simulink model "mophong_quy_dao"  (R2015a)
settings: Solver=ode45  StartTime=0.0  StopTime=322  RelTol=1e-3
values from neighbouring files (symbols this model uses):
  s = [s; t E]    [quydao.m]
undefined symbols (not defined in the file or in its folder): lap, RootGround, RootPart
libraries: mblibv1 x17
settings Model: Creator=Administrator  LastModifiedBy=Administrator
settings SimMechanicsCC: VisOnUpdateDiagram=on  VisDuringSimulation=on

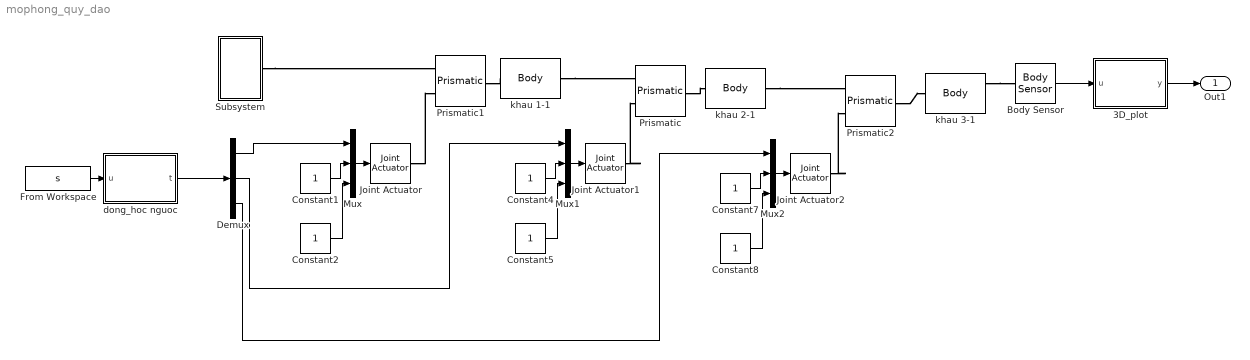
== system mophong_quy_dao ==
  3D_plot : MATLAB Function  TreatAsAtomicUnit=on
  Body Sensor : mblibv1/Sensors &  Actuators/Body Sensor  UpdateFromCAD=off  PhysicalDomain=Mechanical  PortType=blob  Muxed=on  Pose=off  Angle=on  AngleUnits=deg  ArcVelocity=off  ArcVelocityUnits=deg/s  ArcAcceleration=off  ArcAccelerationUnits=deg/s^2  CoordPosition=on  CoordPositionUnits=mm  Velocity=off  VelocityUnits=m/s  Acceleration=off  AccelerationUnits=m/s^2  Quaternion=on  QuaternionDT=off  QuaternionDDT=off  QuaternionUnits=off  OutputVector=[1]  ActiveIO=on  Width=3  DialogClass=MechanicalSensorBlock  ReferenceFrame=Absolute (World)
  Constant{1..2,4..5,7..8} (6 alike) : Constant
  Demux : Demux  Outputs=3
  From Workspace : FromWorkspace  VariableName=s  SampleTime=0.4
  Joint Actuator : mblibv1/Sensors &  Actuators/Joint Actuator  UpdateFromCAD=off  PhysicalDomain=Mechanical  PortType=blob  ActuationStyle=Motion  AngleUnits=deg  ArcVelocityUnits=deg/s  ArcAccelerationUnits=deg/s^2  CoordPositionUnits=mm  VelocityUnits=m/s  AccelerationUnits=m/s^2  ForceUnits=N  TorqueUnits=N*m  ActiveIO=on  Width=3  DialogClass=MechanicalActuatorBlock  Primitive=P1  ReferenceFrame=Absolute (World)
  Joint Actuator1 : mblibv1/Sensors &  Actuators/Joint Actuator  UpdateFromCAD=off  PhysicalDomain=Mechanical  PortType=blob  ActuationStyle=Motion  AngleUnits=deg  ArcVelocityUnits=deg/s  ArcAccelerationUnits=deg/s^2  CoordPositionUnits=mm  VelocityUnits=m/s  AccelerationUnits=m/s^2  ForceUnits=N  TorqueUnits=N*m  ActiveIO=on  Width=3  DialogClass=MechanicalActuatorBlock  Primitive=P1  ReferenceFrame=Absolute (World)
  Joint Actuator2 : mblibv1/Sensors &  Actuators/Joint Actuator  UpdateFromCAD=off  PhysicalDomain=Mechanical  PortType=blob  ActuationStyle=Motion  AngleUnits=deg  ArcVelocityUnits=deg/s  ArcAccelerationUnits=deg/s^2  CoordPositionUnits=mm  VelocityUnits=m/s  AccelerationUnits=m/s^2  ForceUnits=N  TorqueUnits=N*m  ActiveIO=on  Width=3  DialogClass=MechanicalActuatorBlock  Primitive=P1  ReferenceFrame=Absolute (World)
  Mux : Mux  Inputs=3
  Mux1 : Mux  Inputs=3
  Mux2 : Mux  Inputs=3
  Prismatic : mblibv1/Joints/Prismatic  LConnTagsString=__newl0|SA1  RConnTagsString=__newr0  UpdateFromCAD=on  PMImportedID=khau 1-1:-:khau 2-1  NumSAPorts=1  CutJoint=off  MarkAsCut=off  Primitives=prismatic  PrimitiveProps=P1$World$[-1,0,0]$prismatic  DialogClass=JointBlock  P1Axis=[-1,0,0]
  Prismatic1 : mblibv1/Joints/Prismatic  LConnTagsString=__newl0|SA1  RConnTagsString=__newr0  UpdateFromCAD=on  PMImportedID=khau 0-1:-:khau 1-1  NumSAPorts=1  CutJoint=off  MarkAsCut=off  Primitives=prismatic  PrimitiveProps=P1$World$[0,0,1]$prismatic  DialogClass=JointBlock  P1Axis=[0,0,1]
  Prismatic2 : mblibv1/Joints/Prismatic  LConnTagsString=__newl0|SA1  RConnTagsString=__newr0  UpdateFromCAD=on  PMImportedID=khau 2-1:-:khau 3-1  NumSAPorts=1  CutJoint=off  MarkAsCut=off  Primitives=prismatic  PrimitiveProps=P1$World$[0,-1,0]$prismatic  DialogClass=JointBlock  P1Axis=[0,-1,0]
  Subsystem : Subsystem
  dong_hoc nguoc : MATLAB Function  TreatAsAtomicUnit=on
  khau 1-1 : mblibv1/Bodies/Body  LConnTagsString=CS3  RConnTagsString=CS2  UpdateFromCAD=on  PMImportedID=khau 1-1  DialogClass=MechanicalBodyBlock  Mass=0.0250848  MassUnits=kg  InertiaUnits=kg*m^2  Inertia=[0.000583644,0,0;0,0.000587076,0;0,0,3.56803e-05]  Shape=Cylinder  ShapeDims=[1 1]  ShapeUnits=m  ShapeUse=false  Density=1  DensityUnits=kg/m^3  DensityUse=false  GraphicsMode=GFXFILE  GraphicsFileName=lap - khau 1-1.STL  BodyColorSelMode=COLORPALETTE  BodyColor=[0;0.501961;1]  AttachedToCS=CS1  CG=Right$CG$[0.225672 0 0.06]$WORLD$WORLD$m$[0 0 1;-1 0 0;0 -1 0]$3x3 Transform$rad$WORLD$false$khau 1-1::CG(AUTOGEN)  WorkingFrames=Right$CS1$[0 0 0.06]$WORLD$WORLD$m$[0 0 1;-1 0 0;0 -1 0]$3x3 Transform$rad$WORLD$false$khau 1-1::CS1(AUTOGEN)#Right$CS2$[0.48 -0.04 0.1]$WORLD$WORLD$m$[1 0 0;0 1 0;0 0 1]$3x3 Transform$rad$WORLD$true$khau 1-1:-:khau 2-1::khau 1-1(AUTOGEN)#Left$CS3$[-0.05 0.05 0.12]$WORLD$WORLD$m$[1 0 0;0 1 0;0 0 1]$3x3 Transform$rad$WORLD$true$khau 0-1:-:khau 1-1::khau 1-1(AUTOGEN)  CGPos=[0.225672 0 0.06]  CGRot=[0 0 1;-1 0 0;0 -1 0]  CS0Pos=[]  CS0Rot=[]  CS1Pos=[0 0 0.06]  CS1Rot=[0 0 1;-1 0 0;0 -1 0]  CS2Pos=[0.48 -0.04 0.1]  CS2Rot=[1 0 0;0 1 0;0 0 1]  CS3Pos=[-0.05 0.05 0.12]  CS3Rot=[1 0 0;0 1 0;0 0 1]  CS4Pos=[]  CS4Rot=[]  CS5Pos=[]  CS5Rot=[]  CS6Pos=[]  CS6Rot=[]  CS7Pos=[]  CS7Rot=[]  CS8Pos=[]  CS8Rot=[]  CS9Pos=[]  CS9Rot=[]  CS10Pos=[]  CS10Rot=[]  CS11Pos=[]  CS11Rot=[]  CS12Pos=[]  CS12Rot=[]  CS13Pos=[]  CS13Rot=[]  CS14Pos=[]  CS14Rot=[]  CS15Pos=[]  CS15Rot=[]  CS16Pos=[]  CS16Rot=[]  CS17Pos=[]  CS17Rot=[]  CS18Pos=[]  CS18Rot=[]  CS19Pos=[]  CS19Rot=[]  CS20Pos=[]  CS20Rot=[]
  khau 2-1 : mblibv1/Bodies/Body  LConnTagsString=CS2  RConnTagsString=CS3  UpdateFromCAD=on  PMImportedID=khau 2-1  DialogClass=MechanicalBodyBlock  Mass=0.0401856  MassUnits=kg  InertiaUnits=kg*m^2  Inertia=[0.00271366,0,0;0,0.00271765,0;0,0,7.5687e-05]  Shape=Cylinder  ShapeDims=[1 1]  ShapeUnits=m  ShapeUse=false  Density=1  DensityUnits=kg/m^3  DensityUse=false  GraphicsMode=GFXFILE  GraphicsFileName=lap - khau 2-1.STL  BodyColorSelMode=COLORPALETTE  BodyColor=[0.901961;0.709804;0.439216]  AttachedToCS=CS1  CG=Right$CG$[0.42 -0.0425466 0.06]$WORLD$WORLD$m$[0 1 0;0 0 -1;-1 0 0]$3x3 Transform$rad$WORLD$false$khau 2-1::CG(AUTOGEN)  WorkingFrames=Right$CS1$[0.42 0 0.06]$WORLD$WORLD$m$[0 1 0;0 0 -1;-1 0 0]$3x3 Transform$rad$WORLD$false$khau 2-1::CS1(AUTOGEN)#Left$CS2$[0.32 -0.04 0.1]$WORLD$WORLD$m$[1 0 0;0 1 0;0 0 1]$3x3 Transform$rad$WORLD$true$khau 1-1:-:khau 2-1::khau 2-1(AUTOGEN)#Right$CS3$[0.395 -0.06 0.085]$WORLD$WORLD$m$[1 0 0;0 1 0;0 0 1]$3x3 Transform$rad$WORLD$true$khau 2-1:-:khau 3-1::khau 2-1(AUTOGEN)  CGPos=[0.42 -0.0425466 0.06]  CGRot=[0 1 0;0 0 -1;-1 0 0]  CS0Pos=[]  CS0Rot=[]  CS1Pos=[0.42 0 0.06]  CS1Rot=[0 1 0;0 0 -1;-1 0 0]  CS2Pos=[0.32 -0.04 0.1]  CS2Rot=[1 0 0;0 1 0;0 0 1]  CS3Pos=[0.395 -0.06 0.085]  CS3Rot=[1 0 0;0 1 0;0 0 1]  CS4Pos=[]  CS4Rot=[]  CS5Pos=[]  CS5Rot=[]  CS6Pos=[]  CS6Rot=[]  CS7Pos=[]  CS7Rot=[]  CS8Pos=[]  CS8Rot=[]  CS9Pos=[]  CS9Rot=[]  CS10Pos=[]  CS10Rot=[]  CS11Pos=[]  CS11Rot=[]  CS12Pos=[]  CS12Rot=[]  CS13Pos=[]  CS13Rot=[]  CS14Pos=[]  CS14Rot=[]  CS15Pos=[]  CS15Rot=[]  CS16Pos=[]  CS16Rot=[]  CS17Pos=[]  CS17Rot=[]  CS18Pos=[]  CS18Rot=[]  CS19Pos=[]  CS19Rot=[]  CS20Pos=[]  CS20Rot=[]
  khau 3-1 : mblibv1/Bodies/Body  LConnTagsString=CS2  RConnTagsString=CG|CS1  UpdateFromCAD=on  PMImportedID=khau 3-1  DialogClass=MechanicalBodyBlock  Mass=0.00253036  MassUnits=kg  InertiaUnits=kg*m^2  Inertia=[3.10671e-06,0,0;0,4.33218e-06,0;0,0,3.82518e-06]  Shape=Cylinder  ShapeDims=[1 1]  ShapeUnits=m  ShapeUse=false  Density=1  DensityUnits=kg/m^3  DensityUse=false  GraphicsMode=GFXFILE  GraphicsFileName=lap - khau 3-1.STL  BodyColorSelMode=COLORPALETTE  BodyColor=[0.28628 0.66275 0.32941]  AttachedToCS=CS1  CG=Right$CG$[0.416709 -0.66 0.06]$WORLD$WORLD$m$[-1 0 0;0 1 0;0 0 -1]$3x3 Transform$rad$WORLD$true$khau 3-1::CG(AUTOGEN)  WorkingFrames=Right$CS1$[0.31 -0.66 0.06]$WORLD$WORLD$m$[-1 0 0;0 1 0;0 0 -1]$3x3 Transform$rad$WORLD$true$khau 3-1::CS1(AUTOGEN)#Left$CS2$[0.395 -0.72 0.085]$WORLD$WORLD$m$[1 0 0;0 1 0;0 0 1]$3x3 Transform$rad$WORLD$true$khau 2-1:-:khau 3-1::khau 3-1(AUTOGEN)  CGPos=[0.416709 -0.66 0.06]  CGRot=[-1 0 0;0 1 0;0 0 -1]  CS0Pos=[]  CS0Rot=[]  CS1Pos=[0.31 -0.66 0.06]  CS1Rot=[-1 0 0;0 1 0;0 0 -1]  CS2Pos=[0.395 -0.72 0.085]  CS2Rot=[1 0 0;0 1 0;0 0 1]  CS3Pos=[]  CS3Rot=[]  CS4Pos=[]  CS4Rot=[]  CS5Pos=[]  CS5Rot=[]  CS6Pos=[]  CS6Rot=[]  CS7Pos=[]  CS7Rot=[]  CS8Pos=[]  CS8Rot=[]  CS9Pos=[]  CS9Rot=[]  CS10Pos=[]  CS10Rot=[]  CS11Pos=[]  CS11Rot=[]  CS12Pos=[]  CS12Rot=[]  CS13Pos=[]  CS13Rot=[]  CS14Pos=[]  CS14Rot=[]  CS15Pos=[]  CS15Rot=[]  CS16Pos=[]  CS16Rot=[]  CS17Pos=[]  CS17Rot=[]  CS18Pos=[]  CS18Rot=[]  CS19Pos=[]  CS19Rot=[]  CS20Pos=[]  CS20Rot=[]
  Out1 : Outport
  wires:
  Demux/1 -> Mux/1
  Constant1/1 -> Mux/2
  Constant2/1 -> Mux/3
  Mux/1 -> Joint Actuator/1
  Demux/2 -> Mux1/1
  Constant4/1 -> Mux1/2
  Constant5/1 -> Mux1/3
  Mux1/1 -> Joint Actuator1/1
  Demux/3 -> Mux2/1
  Constant7/1 -> Mux2/2
  Constant8/1 -> Mux2/3
  Mux2/1 -> Joint Actuator2/1
  dong_hoc nguoc/1(t) -> Demux/1
  Body Sensor/1 -> 3D_plot/1(u)
  3D_plot/1(y) -> Out1/1
  From Workspace/1 -> dong_hoc nguoc/1(u)
  connections:
  khau 1-1/RConn1 -- Prismatic/LConn1
  Prismatic/RConn1 -- khau 2-1/LConn1
  Prismatic1/RConn1 -- khau 1-1/LConn1
  khau 2-1/RConn1 -- Prismatic2/LConn1
  Prismatic2/RConn1 -- khau 3-1/LConn1
  Joint Actuator/RConn1 -- Prismatic1/LConn2
  Joint Actuator1/RConn1 -- Prismatic/LConn2
  Joint Actuator2/RConn1 -- Prismatic2/LConn2
  khau 3-1/RConn1 -- Body Sensor/LConn1
  Subsystem/RConn1 -- Prismatic1/LConn1

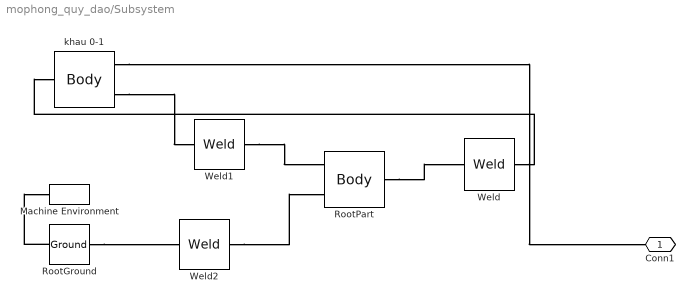
== system mophong_quy_dao/Subsystem ==
  Machine Environment : mblibv1/Bodies/Machine Environment  PortType=env  PhysicalDomain=Mechanical  DialogTemplateClass=MECH.MachineEnvironment  SyncWhenCopied=off  Gravity=[0 -9.81 0]  GravityUnits=m/s^2  GravityAsSignal=off  Dimensionality=Auto-detect  AnalysisType=Forward dynamics  LinearAssemblyTolerance=1e-3  LinearAssemblyToleranceUnits=m  AngularAssemblyTolerance=1e-3  AngularAssemblyToleranceUnits=rad  ConstraintSolverType=Stabilizing  ConstraintRelTolerance=1e-4  ConstraintAbsTolerance=1e-4  UseRobustSingularityHandling=off  RedundancyAnalysisToleranceType=Automatically select tolerance  RedundancyAnalysisTolerance=1e-14  StatePerturbationType=Fixed  PerturbationSize=1e-5  VisualizeMachine=on  BodyVisualizationType=Use model default body geometries  BodyColorSelMode=Use model default  DefaultBodyColor=[1 0 0]
  RootGround : mblibv1/Bodies/Ground  UpdateFromCAD=on  PMImportedID=RootGround  LeftPortType=env  RightPortType=workingframe  PhysicalDomain=Mechanical  DialogClass=GroundBlock  CoordPosition=[0.0188363,-0.0133914,0.352544]  CoordPositionUnits=m  StateVectorMgrId=0  MachineId=[1 0]  ShowEnvPort=on  ParameterChecksum=[2388317299, 529211876, 2012815551, 1180572592]  TopologyChecksum=[3572386912, 2938984299, 652651862, 2599928849]
  RootPart : mblibv1/Bodies/Body  LConnTagsString=CS3|CS4  RConnTagsString=CS2  UpdateFromCAD=on  PMImportedID=lap/RootPart  DialogClass=MechanicalBodyBlock  Mass=0  MassUnits=kg  InertiaUnits=kg*m^2  Inertia=[0,0,0;0,0,0;0,0,0]  Shape=Cylinder  ShapeDims=[1 1]  ShapeUnits=m  ShapeUse=false  Density=1  DensityUnits=kg/m^3  DensityUse=false  GraphicsMode=MACHINE_DEFAULT  BodyColorSelMode=MACHINE_DEFAULT  BodyColor=[1;0;0]  AttachedToCS=CS1  CG=Right$CG$[0.0188363 -0.0133914 0.352544]$WORLD$WORLD$m$[1 0 0;0 1 0;0 0 1]$3x3 Transform$rad$WORLD$false$lap/RootPart::CG(AUTOGEN)  WorkingFrames=Right$CS1$[0 0 0]$WORLD$WORLD$m$[1 0 0;0 1 0;0 0 1]$3x3 Transform$rad$WORLD$false$lap/RootPart::CS1(AUTOGEN)#Right$CS2$[-0.102063 0 0.46]$WORLD$WORLD$m$[1 0 0;0 1 0;0 0 1]$3x3 Transform$rad$WORLD$true$khau 0-1:-:lap/RootPart::lap/RootPart(AUTOGEN)#Left$CS3$[-0.102063 0 0.46]$WORLD$WORLD$m$[1 0 0;0 1 0;0 0 1]$3x3 Transform$rad$WORLD$true$:-:khau 0-1::lap/RootPart(AUTOGEN)#Left$CS4$[0.0188363 -0.0133914 0.352544]$WORLD$WORLD$m$[1 0 0;0 1 0;0 0 1]$3x3 Transform$rad$WORLD$true$RootGround:-:lap/RootPart::lap/RootPart(AUTOGEN)  CGPos=[0.0188363 -0.0133914 0.352544]  CGRot=[1 0 0;0 1 0;0 0 1]  CS0Pos=[]  CS0Rot=[]  CS1Pos=[0 0 0]  CS1Rot=[1 0 0;0 1 0;0 0 1]  CS2Pos=[-0.102063 0 0.46]  CS2Rot=[1 0 0;0 1 0;0 0 1]  CS3Pos=[-0.102063 0 0.46]  CS3Rot=[1 0 0;0 1 0;0 0 1]  CS4Pos=[0.0188363 -0.0133914 0.352544]  CS4Rot=[1 0 0;0 1 0;0 0 1]  CS5Pos=[]  CS5Rot=[]  CS6Pos=[]  CS6Rot=[]  CS7Pos=[]  CS7Rot=[]  CS8Pos=[]  CS8Rot=[]  CS9Pos=[]  CS9Rot=[]  CS10Pos=[]  CS10Rot=[]  CS11Pos=[]  CS11Rot=[]  CS12Pos=[]  CS12Rot=[]  CS13Pos=[]  CS13Rot=[]  CS14Pos=[]  CS14Rot=[]  CS15Pos=[]  CS15Rot=[]  CS16Pos=[]  CS16Rot=[]  CS17Pos=[]  CS17Rot=[]  CS18Pos=[]  CS18Rot=[]  CS19Pos=[]  CS19Rot=[]  CS20Pos=[]  CS20Rot=[]
  Weld : mblibv1/Joints/Weld  LConnTagsString=__newl0  RConnTagsString=__newr0  UpdateFromCAD=on  PMImportedID=khau 0-1:-:lap/RootPart  NumSAPorts=0  CutJoint=off  MarkAsCut=off  Primitives=weld  PrimitiveProps=W$World$[0.57735,0.57735,0.57735]$weld  DialogClass=JointBlock  WAxis=[0.57735,0.57735,0.57735]
  Weld1 : mblibv1/Joints/Weld  LConnTagsString=__newl0  RConnTagsString=__newr0  UpdateFromCAD=on  PMImportedID=:-:khau 0-1  NumSAPorts=0  CutJoint=off  MarkAsCut=off  Primitives=weld  PrimitiveProps=W$WORLD$[0.57735,0.57735,0.57735]$weld  DialogClass=JointBlock  WAxis=[0.57735,0.57735,0.57735]
  Weld2 : mblibv1/Joints/Weld  LConnTagsString=__newl0  RConnTagsString=__newr0  UpdateFromCAD=on  PMImportedID=RootGround:-:lap/RootPart  NumSAPorts=0  CutJoint=off  MarkAsCut=off  Primitives=weld  PrimitiveProps=W$WORLD$[0.57735,0.57735,0.57735]$weld  DialogClass=JointBlock  WAxis=[0.57735,0.57735,0.57735]
  khau 0-1 : mblibv1/Bodies/Body  LConnTagsString=CS2  RConnTagsString=CS3|CS4  UpdateFromCAD=on  PMImportedID=khau 0-1  DialogClass=MechanicalBodyBlock  Mass=0.184586  MassUnits=kg  InertiaUnits=kg*m^2  Inertia=[0.0366621,0,0;0,0.0391956,0;0,0,0.0032657]  Shape=Cylinder  ShapeDims=[1 1]  ShapeUnits=m  ShapeUse=false  Density=1  DensityUnits=kg/m^3  DensityUse=false  GraphicsMode=GFXFILE  GraphicsFileName=lap - khau 0-1.STL  BodyColorSelMode=COLORPALETTE  BodyColor=[1;1;0]  AttachedToCS=CS1  CG=Right$CG$[-0.102063 0 0.46]$WORLD$WORLD$m$[1 0 0;0 1 0;0 0 1]$3x3 Transform$rad$WORLD$false$khau 0-1::CG(AUTOGEN)  WorkingFrames=Right$CS1$[0 0 0]$WORLD$WORLD$m$[1 0 0;0 1 0;0 0 1]$3x3 Transform$rad$WORLD$false$khau 0-1::CS1(AUTOGEN)#Left$CS2$[-0.102063 0 0.46]$WORLD$WORLD$m$[1 0 0;0 1 0;0 0 1]$3x3 Transform$rad$WORLD$true$khau 0-1:-:lap/RootPart::khau 0-1(AUTOGEN)#Right$CS3$[-0.05 0.05 0.92]$WORLD$WORLD$m$[1 0 0;0 1 0;0 0 1]$3x3 Transform$rad$WORLD$true$khau 0-1:-:khau 1-1::khau 0-1(AUTOGEN)#Right$CS4$[-0.102063 0 0.46]$WORLD$WORLD$m$[1 0 0;0 1 0;0 0 1]$3x3 Transform$rad$WORLD$true$:-:khau 0-1::khau 0-1(AUTOGEN)  CGPos=[-0.102063 0 0.46]  CGRot=[1 0 0;0 1 0;0 0 1]  CS0Pos=[]  CS0Rot=[]  CS1Pos=[0 0 0]  CS1Rot=[1 0 0;0 1 0;0 0 1]  CS2Pos=[-0.102063 0 0.46]  CS2Rot=[1 0 0;0 1 0;0 0 1]  CS3Pos=[-0.05 0.05 0.92]  CS3Rot=[1 0 0;0 1 0;0 0 1]  CS4Pos=[-0.102063 0 0.46]  CS4Rot=[1 0 0;0 1 0;0 0 1]  CS5Pos=[]  CS5Rot=[]  CS6Pos=[]  CS6Rot=[]  CS7Pos=[]  CS7Rot=[]  CS8Pos=[]  CS8Rot=[]  CS9Pos=[]  CS9Rot=[]  CS10Pos=[]  CS10Rot=[]  CS11Pos=[]  CS11Rot=[]  CS12Pos=[]  CS12Rot=[]  CS13Pos=[]  CS13Rot=[]  CS14Pos=[]  CS14Rot=[]  CS15Pos=[]  CS15Rot=[]  CS16Pos=[]  CS16Rot=[]  CS17Pos=[]  CS17Rot=[]  CS18Pos=[]  CS18Rot=[]  CS19Pos=[]  CS19Rot=[]  CS20Pos=[]  CS20Rot=[]
  Conn1 : PMIOPort  Port=1  Side=Right
  connections:
  RootPart/RConn1 -- Weld/LConn1
  Weld/RConn1 -- khau 0-1/LConn1
  khau 0-1/RConn1 -- Conn1/RConn1
  khau 0-1/RConn2 -- Weld1/LConn1
  Weld1/RConn1 -- RootPart/LConn1
  RootGround/RConn1 -- Weld2/LConn1
  Weld2/RConn1 -- RootPart/LConn2
  RootGround/LConn1 -- Machine Environment/RConn1

== matlab function mophong_quy_dao/3D_plot ==
  data: u input; y output
function y = fcn(u)
%#codegen
x1=u(1,1)
x2=u(2,1)
x3=u(3,1)
plot3(-x3,x2,x1,'b.');
hold on;
grid on
y = u;

== matlab function mophong_quy_dao/dong_hoc nguoc ==
  data: u input; t output
function t = fcn(u)
%#codegen
x=u(1);
y=u(2);
z=u(3);
vx=u(4);
vy=u(5);
vz=u(6);
ax=u(7);
ay=u(8);
az=u(9)
d1=60;
d2=360;
d3=620;
a3=110;
t1=z-d1;
t2=-x+d2-a3;
t3=-y-d3;

t1_dot=vz;
t2_dot=-vx;
t3_dot=-vy;

t1_2dot=az;
t2_2dot=-ax;
t3_2dot=-ay;
t=[t1 t2 t3 ]
